simulink model "exnb4137986_Q7"  (R2023b)
settings: Solver=FixedStepAuto  StartTime=0.0  StopTime=5  FixedStep=0.001  RelTol=1e-3
values from neighbouring files (symbols this model uses):
  K = place(A, B, lambda_cl)    [exnb4137986_Q10_par.m]    (also in exnb4137986_Q7_par.m; exnb4137986_Q8_par.m; exnb4137986_Q9_par.m)
  N_bar = N_u + K * N_x    [exnb4137986_Q7_par.m]
  values = [0, 0.01, 1, 0.001, 1, 1, 10]    [exnb4137986_Q10_par.m]    (also in exnb4137986_Q4_par.m; exnb4137986_Q5_par.m; exnb4137986_Q7_par.m; exnb4137986_Q8_par.m)
  x_star_1 = [I_star_1, omega_star_1]    [exnb4137986_Q10_par.m]    (also in exnb4137986_Q4_par.m = [omega_star_1, I_star_1]; exnb4137986_Q5_par.m; exnb4137986_Q7_par.m; exnb4137986_Q8_par.m)
  x_star_2 = [0, 10]    [exnb4137986_Q10_par.m]    (also in exnb4137986_Q7_par.m; exnb4137986_Q8_par.m)
  x_star_3 = [0, 0]    [exnb4137986_Q10_par.m]    (also in exnb4137986_Q7_par.m)
settings Model: Creator=therkelsen  LastModifiedBy=therkelsen
settings RTWCC: GPUComputeCapability=5.0

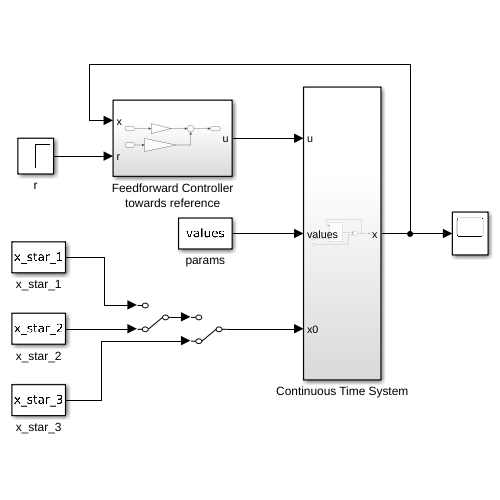
[thumbnail: Simulink's stored preview of the top-level diagram]
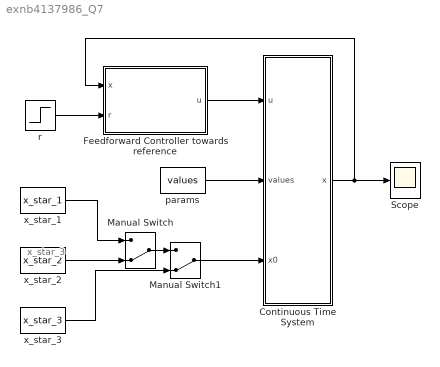
== system exnb4137986_Q7 ==
  note: x_star_3
  Continuous Time System : Subsystem
  Feedforward Controller towards reference : Subsystem
  Manual Switch : ManualSwitch  CurrentSetting=0
  Manual Switch1 : ManualSwitch  CurrentSetting=0
  Scope : Scope
  params : Constant  Value=values
  r : Step  After=20  SampleTime=0
  x_star_1 : Constant  Value=x_star_1
  x_star_2 : Constant  Value=x_star_2
  x_star_3 : Constant  Value=x_star_3
  wires:
  Continuous Time System/1(x) -> Feedforward Controller towards reference/1(x), Scope/1
  Manual Switch1/1 -> Continuous Time System/3(x0)
  Feedforward Controller towards reference/1(u) -> Continuous Time System/1(u)
  params/1 -> Continuous Time System/2(values)
  x_star_2/1 -> Manual Switch/2
  x_star_1/1 -> Manual Switch/1
  r/1 -> Feedforward Controller towards reference/2(r)
  x_star_3/1 -> Manual Switch1/2
  Manual Switch/1 -> Manual Switch1/1

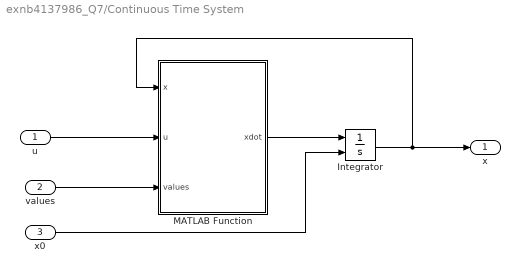
== system exnb4137986_Q7/Continuous Time System ==
  u : Inport
  values : Inport  Port=2
  x0 : Inport  Port=3
  Integrator : Integrator  InitialConditionSource=external
  MATLAB Function : MATLAB Function  TreatAsAtomicUnit=on
  x : Outport
  wires:
  MATLAB Function/1(xdot) -> Integrator/1
  values/1 -> MATLAB Function/3(values)
  u/1 -> MATLAB Function/2(u)
  Integrator/1 -> x/1, MATLAB Function/1(x)
  x0/1 -> Integrator/2

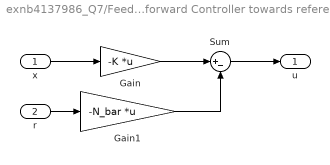
== system exnb4137986_Q7/Feedforward Controller towards reference ==
  x : Inport
  r : Inport  Port=2
  Gain : Gain  Gain=-K  Multiplication=Matrix(K*u)
  Gain1 : Gain  Gain=-N_bar  Multiplication=Matrix(K*u) (u vector)
  Sum : Sum  Inputs=|+-
  u : Outport
  wires:
  x/1 -> Gain/1
  r/1 -> Gain1/1
  Sum/1 -> u/1
  Gain/1 -> Sum/1
  Gain1/1 -> Sum/2

== matlab function exnb4137986_Q7/Continuous Time System/MATLAB Function ==
  data: x input; u input; xdot output; values input
function xdot = fcn(x, u, values)

J = values(2);
L = values(3);
Kd = values(4);
Ke = values(5);
Km = values(6);
Rm = values(7);

xdot = [-Rm/L * x(1) - Ke/L * x(2) + 1/L * u;
         Km/J * x(1) - Kd/J * x(2)];
